simulink model "high_frequency"  (R2023a)
settings: Solver=VariableStepAuto  StartTime=0.0  StopTime=10.0  RelTol=1e-3
settings Model: Creator=belov  LastModifiedBy=belov

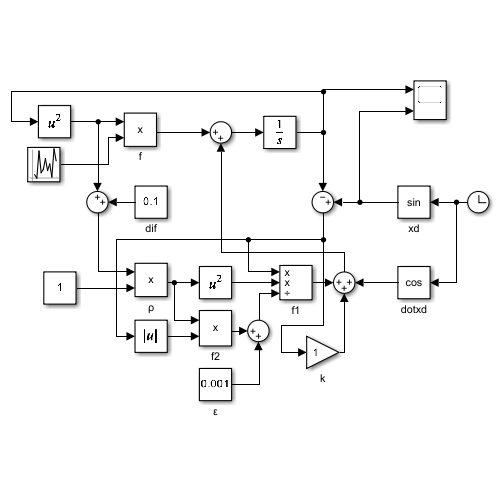
[thumbnail: Simulink's stored preview of the top-level diagram]
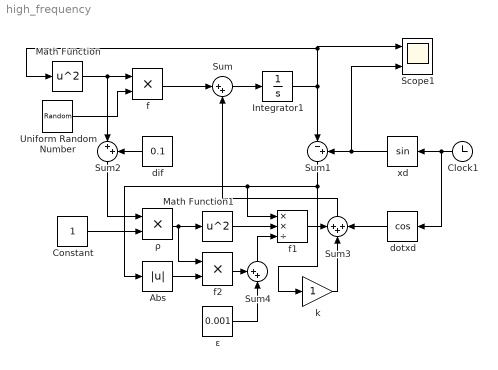
== system high_frequency ==
  Abs : Abs  SaturateOnIntegerOverflow=off
  Clock1 : Clock
  Constant : Constant
  Integrator1 : Integrator  InitialCondition=1
  Math Function : Math  Operator=square
  Math Function1 : Math  Operator=square
  Scope1 : Scope  NumInputPorts=2
  Sum : Sum  Inputs=|++
  Sum1 : Sum  Inputs=|-+
  Sum2 : Sum  Inputs=|++
  Sum3 : Sum  Inputs=+++
  Sum4 : Sum  Inputs=++|
  Uniform Random Number : UniformRandomNumber  SampleTime=0.1
  dif : Constant  Value=0.1
  dotxd : Trigonometry  Operator=cos
  f : Product  Inputs=**
  f1 : Product  Inputs=**/
  f2 : Product  Inputs=**
  k : Gain
  xd : Trigonometry
  ε : Constant  Value=0.001
  ρ : Product  Inputs=**
  wires:
  Sum1/1 -> k/1, f1/1, Abs/1
  Clock1/1 -> dotxd/1, xd/1
  Constant/1 -> ρ/2
  ρ/1 -> f2/1, Math Function1/1
  k/1 -> Sum3/2
  Sum2/1 -> ρ/1
  f1/1 -> Sum3/1
  dif/1 -> Sum2/2
  Sum3/1 -> Sum/2
  xd/1 -> Scope1/2, Sum1/2
  Math Function/1 -> f/1, Sum2/1
  dotxd/1 -> Sum3/3
  Sum/1 -> Integrator1/1
  Math Function1/1 -> f1/2
  Uniform Random Number/1 -> f/2
  Integrator1/1 -> Sum1/1, Math Function/1, Scope1/1
  f/1 -> Sum/1
  Abs/1 -> f2/2
  Sum4/1 -> f1/3
  f2/1 -> Sum4/1
  ε/1 -> Sum4/2
